simulink model "quy_dao_2diem_5lan"  (R2022b)
settings: Solver=FixedStepAuto  StartTime=0.0  StopTime=10.0  FixedStep=0.01  RelTol=1e-3
settings Model: Creator=Admin  LastModifiedBy=Admin

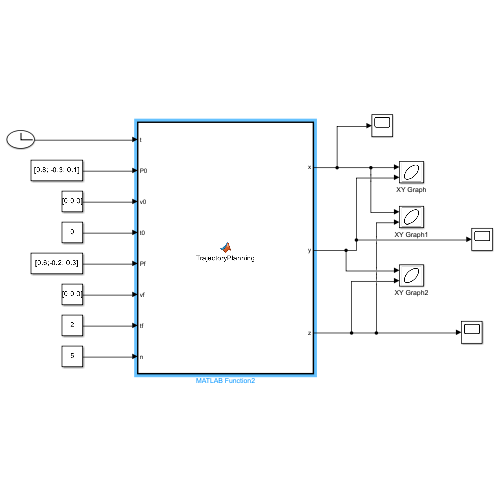
[thumbnail: Simulink's stored preview of the top-level diagram]
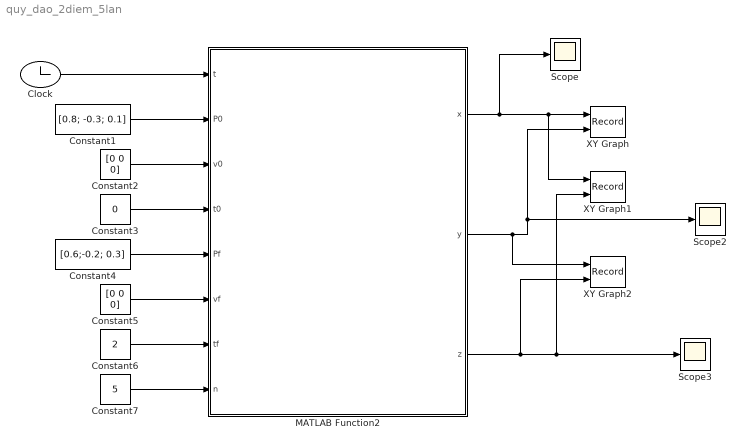
== system quy_dao_2diem_5lan ==
  Clock : Clock
      settings: Decimation=20
  Constant1 : Constant  Value=[0.8; -0.3; 0.1]
  Constant2 : Constant  Value=[0 0 0]
  Constant3 : Constant  Value=0
  Constant4 : Constant  Value=[0.6;-0.2; 0.3]
  Constant5 : Constant  Value=[0 0 0]
  Constant6 : Constant  Value=2
  Constant7 : Constant  Value=5
  MATLAB Function2 : MATLAB Function  TreatAsAtomicUnit=on
  Scope : Scope
  Scope2 : Scope
  Scope3 : Scope
  XY Graph : Record  FileSettingsInternal="{\"entries\":[{\"content\":{\"excelSettings\":{\"content\":{},\"type\":\"Streamout.ExcelSettings\"}},\"type\":\"Streamout.FileSettingStorage\",\"uuid\":\"603df023-5dc1-4a77-802f-1d359ca11c91\"}],\"packageUris\":[\"http://schema.mathworks.com/mf0/streamout_blocks/R2020a\"],\"version\":\"1.0\"}"  Layout=[1 1]  SignalsInternal="{\"entries\":[{\"content\":{\"signals\":[{\"content\":{\"blockPath\":[\"quy_dao_2diem_5lan/XY Graph\"],\"channel\":[],\"dimensions\":[1],\"domain\":\"quy_dao_2diem_5lan/XY Graph\",\"lineColor\":\"#a2142f\",\"plots\":[1],\"port\":1,\"sid\":[\"\"],\"signalID\":1151,\"signalName\":\"MATLAB Function2:1\"},\"type\":\"RecordBlkView.Signal\",\"uuid\":\"a780c1dd-2385-4ba4-a495-f8dc50ceeb4a\"},{\"content\":{\"blockPath\":[\"quy_dao_2diem_5lan/XY Graph\"],\"channel\":[],\"dimensions\":[1],\"domain\":\"quy_dao_2diem_5lan/XY Graph\",\"lineColor\":\"#139fff\",\"plots\":[1],\"port\":2,\"sid\":[\"\"],\"signalID\":1155,\"signalName\":\"MATLAB Function2:2\"},\"type\":\"RecordBlkView.Signal\",\"uuid\":\"2caabff1-c474-4b8f-964c-32a5460fb7b2\"}]},\"type\":\"RecordBlkView.InputSignals\",\"uuid\":\"d5347b53-71af-4bff-8b37-8af6bf656f73\"}],\"packageUris\":[\"http://schema.mathworks.com/mf0/streamout_blocks/R2020a\"],\"version\":\"1.0\"}"  VisualizationBindings="{\"xyplotplugin\":{\"info\":[{\"series\":[{\"bindingParametersList\":[{\"parameter\":\"X-Axis\",\"signalID\":1151,\"signalName\":\"MATLAB Function2:1\"},{\"parameter\":\"Y-Axis\",\"signalID\":1155,\"signalName\":\"MATLAB Function2:2\"}],\"seriesID\":26285}],\"subplotID\":1}]}}"  CompatibilityTag=XY
  XY Graph1 : Record  FileSettingsInternal="{\"entries\":[{\"content\":{\"excelSettings\":{\"content\":{},\"type\":\"Streamout.ExcelSettings\"}},\"type\":\"Streamout.FileSettingStorage\",\"uuid\":\"80f93ef0-56c1-49dd-9e7d-a9e540be2e63\"}],\"packageUris\":[\"http://schema.mathworks.com/mf0/streamout_blocks/R2020a\"],\"version\":\"1.0\"}"  Layout=[1 1]  SignalsInternal="{\"entries\":[{\"content\":{\"signals\":[{\"content\":{\"blockPath\":[\"quy_dao_2diem_5lan/XY Graph1\"],\"channel\":[],\"dimensions\":[1],\"domain\":\"quy_dao_2diem_5lan/XY Graph1\",\"lineColor\":\"#a2142f\",\"plots\":[1],\"port\":1,\"sid\":[\"\"],\"signalID\":1159,\"signalName\":\"MATLAB Function2:1\"},\"type\":\"RecordBlkView.Signal\",\"uuid\":\"4132f046-dd83-4136-85bd-46de1661bea8\"},{\"content\":{\"blockPath\":[\"quy_dao_2diem_5lan/XY Graph1\"],\"channel\":[],\"dimensions\":[1],\"domain\":\"quy_dao_2diem_5lan/XY Graph1\",\"lineColor\":\"#139fff\",\"plots\":[1],\"port\":2,\"sid\":[\"\"],\"signalID\":1163,\"signalName\":\"MATLAB Function2:3\"},\"type\":\"RecordBlkView.Signal\",\"uuid\":\"73bf966e-22e0-4740-b982-598efa7be928\"}]},\"type\":\"RecordBlkView.InputSignals\",\"uuid\":\"41e4ed72-2c4c-4019-aa2a-300eb3ee5ce7\"}],\"packageUris\":[\"http://schema.mathworks.com/mf0/streamout_blocks/R2020a\"],\"version\":\"1.0\"}"  VisualizationBindings="{\"xyplotplugin\":{\"info\":[{\"series\":[{\"bindingParametersList\":[{\"parameter\":\"X-Axis\",\"signalID\":1159,\"signalName\":\"MATLAB Function2:1\"},{\"parameter\":\"Y-Axis\",\"signalID\":1163,\"signalName\":\"MATLAB Function2:3\"}],\"seriesID\":22230}],\"subplotID\":1}]}}"  CompatibilityTag=XY
  XY Graph2 : Record  FileSettingsInternal="{\"entries\":[{\"content\":{\"excelSettings\":{\"content\":{},\"type\":\"Streamout.ExcelSettings\"}},\"type\":\"Streamout.FileSettingStorage\",\"uuid\":\"69a53295-0371-4d9e-84a1-12216b985ff9\"}],\"packageUris\":[\"http://schema.mathworks.com/mf0/streamout_blocks/R2020a\"],\"version\":\"1.0\"}"  Layout=[1 1]  SignalsInternal="{\"entries\":[{\"content\":{\"signals\":[{\"content\":{\"blockPath\":[\"quy_dao_2diem_5lan/XY Graph2\"],\"channel\":[],\"dimensions\":[1],\"domain\":\"quy_dao_2diem_5lan/XY Graph2\",\"lineColor\":\"#a2142f\",\"plots\":[1],\"port\":1,\"sid\":[\"\"],\"signalID\":1167,\"signalName\":\"MATLAB Function2:2\"},\"type\":\"RecordBlkView.Signal\",\"uuid\":\"6008df6b-b169-4e51-a00d-a5806cc5c458\"},{\"content\":{\"blockPath\":[\"quy_dao_2diem_5lan/XY Graph2\"],\"channel\":[],\"dimensions\":[1],\"domain\":\"quy_dao_2diem_5lan/XY Graph2\",\"lineColor\":\"#139fff\",\"plots\":[1],\"port\":2,\"sid\":[\"\"],\"signalID\":1171,\"signalName\":\"MATLAB Function2:3\"},\"type\":\"RecordBlkView.Signal\",\"uuid\":\"60be858b-8975-4221-a6a4-2384ab84b649\"}]},\"type\":\"RecordBlkView.InputSignals\",\"uuid\":\"6878b731-d69f-4365-a4d2-c90a58ee6107\"}],\"packageUris\":[\"http://schema.mathworks.com/mf0/streamout_blocks/R2020a\"],\"version\":\"1.0\"}"  VisualizationBindings="{\"xyplotplugin\":{\"info\":[{\"series\":[{\"bindingParametersList\":[{\"parameter\":\"X-Axis\",\"signalID\":1167,\"signalName\":\"MATLAB Function2:2\"},{\"parameter\":\"Y-Axis\",\"signalID\":1171,\"signalName\":\"MATLAB Function2:3\"}],\"seriesID\":44429}],\"subplotID\":1}]}}"  CompatibilityTag=XY
  wires:
  Clock/1 -> MATLAB Function2/1(t)
  Constant1/1 -> MATLAB Function2/2(P0)
  Constant2/1 -> MATLAB Function2/3(v0)
  Constant3/1 -> MATLAB Function2/4(t0)
  Constant4/1 -> MATLAB Function2/5(Pf)
  Constant5/1 -> MATLAB Function2/6(vf)
  Constant6/1 -> MATLAB Function2/7(tf)
  Constant7/1 -> MATLAB Function2/8(n)
  MATLAB Function2/1(x) -> Scope/1, XY Graph1/1, XY Graph/1
  MATLAB Function2/2(y) -> XY Graph2/1, Scope2/1, XY Graph/2
  MATLAB Function2/3(z) -> XY Graph2/2, XY Graph1/2, Scope3/1

== matlab function quy_dao_2diem_5lan/MATLAB Function2 ==
  data: t input; x output; y output; P0 input; v0 input; t0 input; Pf input; vf input; tf input; n input; z output
function [x,y,z] = TrajectoryPlanning(t,P0,v0,t0,Pf,vf,tf,n)
a10_AB=P0(1);
a20_AB=P0(2);
a30_AB=P0(3);
a11_AB=v0(1);
a21_AB=v0(2);
a31_AB=v0(3);
a12_AB=3/(tf-t0)^2*(Pf(1)-P0(1))-2/(tf-t0)*v0(1)-1/(tf-t0)*vf(1);
a22_AB=3/(tf-t0)^2*(Pf(2)-P0(2))-2/(tf-t0)*v0(2)-1/(tf-t0)*vf(2);
a32_AB=3/(tf-t0)^2*(Pf(3)-P0(3))-2/(tf-t0)*v0(3)-1/(tf-t0)*vf(3);
a13_AB=-2/(tf-t0)^3*(Pf(1)-P0(1))+1/(tf-t0)^2*(vf(1)+v0(1));
a23_AB=-2/(tf-t0)^3*(Pf(2)-P0(2))+1/(tf-t0)^2*(vf(2)+v0(2));
a33_AB=-2/(tf-t0)^3*(Pf(3)-P0(3))+1/(tf-t0)^2*(vf(3)+v0(3));

 
a10_BA=Pf(1);
a20_BA=Pf(2);
a30_BA=Pf(3);
a11_BA=vf(1);
a21_BA=vf(2);
a31_BA=vf(3);
a12_BA=3/(t0-tf)^2*(P0(1)-Pf(1))-2/(t0-tf)*vf(1)-1/(t0-tf)*v0(1);
a22_BA=3/(t0-tf)^2*(P0(2)-Pf(2))-2/(t0-tf)*vf(2)-1/(t0-tf)*v0(2);
a32_BA=3/(t0-tf)^2*(P0(3)-Pf(3))-2/(t0-tf)*vf(3)-1/(t0-tf)*v0(3);
a13_BA=2/(t0-tf)^3*(P0(1)-Pf(1))+1/(t0-tf)^2*(v0(1)+vf(1));
a23_BA=2/(t0-tf)^3*(P0(2)-Pf(2))+1/(t0-tf)^2*(v0(2)+vf(2));
a33_BA=2/(t0-tf)^3*(P0(3)-Pf(3))+1/(t0-tf)^2*(v0(3)+vf(3));

 
i=fix(t/tf);

if (rem(i,2)==1)&&(i<(n*2 + 1))
      tt=t-tf*i;
      x=a10_AB+a11_AB*tt+a12_AB*tt^2+a13_AB*tt^3;
      y=a20_AB+a21_AB*tt+a22_AB*tt^2+a23_AB*tt^3;
      z=a30_AB+a31_AB*tt+a32_AB*tt^2+a33_AB*tt^3;
      plot3(x,y,z,'.');
      hold on
elseif (rem(i,2)==0)&&(i<(n*2 + 1))
      tt=t-tf*i;
      x=a10_BA+a11_BA*tt+a12_BA*tt^2+a13_BA*tt^3;
      y=a20_BA+a21_BA*tt+a22_BA*tt^2+a23_BA*tt^3;
      z=a30_BA+a31_BA*tt+a32_BA*tt^2+a33_BA*tt^3;
      plot3(x,y,z,'.');
      hold on
else
      x=P0(1);
      y=P0(2);
      z=P0(3);
      plot3(x,y,z,'.');
      hold on
end
